simulink model "schema_simple"  (Simulink 7.0)
settings: Solver=ode5  SolverMode=SingleTasking  StartTime=0.0  StopTime=Inf  FixedStep=1e-3  MaxStep=0.001  RelTol=1e-3  AbsTol=1e-5
PreLoadFcn:
  | Ts=1e-3;
  | zdroj = 1;
  | man_w = 0.5
PostLoadFcn:
  | if ~exist('dsparch4','file') errordlg('Signal Processing Blockset is required to run this demo.', 'Signal Processing Blockset required'); end
undefined symbols (not defined in the file): Humusoft, MF624
libraries: rtwinlib x2
settings Model: Creator=Sehnal  SimulationMode=external  CovMetricSettings=d  ExtModeTrigDuration=50000  ExtModeTrigLevel=0.500000  ExtModeAutoUpdateStatusClock=off
settings SolverCC: PositivePriorityOrder=on
settings DataIOCC: LimitDataPoints=off  MaxDataPoints=10000  SaveOutput=off  SignalLogging=off  SaveTime=off  SignalLoggingName=logsOut
settings OptimizationCC: BooleanDataType=off
settings DebuggingCC: SaveWithParameterizedLinksMsg=none  CheckExecutionContextPreStartOutputMsg=on  CheckExecutionContextRuntimeOutputMsg=on  SignalResolutionControl=TryResolveAllWithWarning  SolverPrmCheckMsg=none  MultiTaskDSMMsg=warning  MultiTaskCondExecSysMsg=none  StrictBusMsg=None
settings HardwareCC: TargetEndianess=LittleEndian  TargetHWDeviceType=MATLAB Host  ProdEqTarget=off
settings ModelReferenceCC: UpdateModelReferenceTargets=IfOutOfDate  ModelReferenceNumInstancesAllowed=Zero
settings RTWCC: SystemTargetFile=rtwin.tlc  TemplateMakefile=rtwin.tmf  RetainRTWFile=on  ProcessScript=rtwin_make_rtw_hook  IncludeERTFirstTime=on
settings RTWinTargetCC: TargetFcnLib=ansi_tfl_tmw.mat  GenFloatMathFcnCalls=ANSI_C  ModelReferenceCompliant=off  CompOptLevelCompliant=off  PortableWordSizes=off  CCOptimize=on

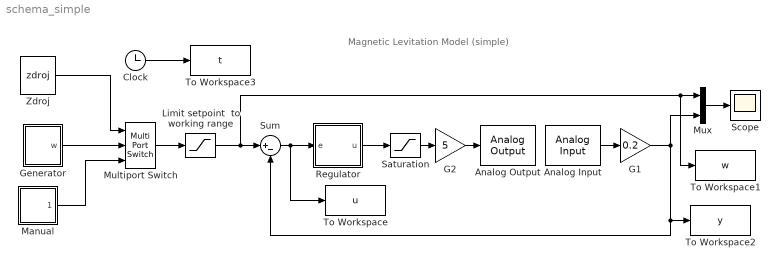
== system schema_simple ==
  note: Magnetic Levitation Model
      | (simple)
  Analog Input : rtwinlib/Analog Input  SampleTime=1e-3  DrvName=Humusoft/MF624  DrvAddress=4294967295  DrvOptions=0  Channels=1  RangeMode=1  VoltRange=1  DataType=1
      settings: AttributesFormatString=Humusoft\nMF624 [auto]
  Analog Output : rtwinlib/Analog Output  SampleTime=1e-3  DrvName=Humusoft/MF624  DrvAddress=4294967295  DrvOptions=0  Channels=1  RangeMode=1  VoltRange=1  InitialValue=0  FinalValue=0
      settings: AttributesFormatString=Humusoft\nMF624 [auto]
  Clock : Clock
      settings: Decimation=10
  G1 : Gain  Gain=0.2  ParameterDataType=sfix(16)  ParameterScaling=2^0  OutDataType=sfix(16)  OutScaling=2^0  SaturateOnIntegerOverflow=on
  G2 : Gain  Gain=5  ParameterDataType=sfix(16)  ParameterScaling=2^0  OutDataType=sfix(16)  OutScaling=2^0  SaturateOnIntegerOverflow=on
  Generator : Subsystem
  "Limit setpoint  to working range  " : Saturate  UpperLimit=0.8  LowerLimit=0  ZeroCross=off
  Manual : Subsystem
  Multiport Switch : MultiPortSwitch  Inputs=2
  Mux : Mux  Inputs=2
  Regulator : Subsystem
  Saturation : Saturate  UpperLimit=1  LowerLimit=0  ZeroCross=off
  Scope : Scope
      settings: TimeRange=5  YMin=-0.05  YMax=0.95  SaveName=last  DataFormat=Array  MaxDataPoints=1  SampleInput=on  SampleTime=0.02
  Sum : Sum  Inputs=|+-  OutDataType=sfix(16)  OutScaling=2^0  SaturateOnIntegerOverflow=on  InputSameDT=on
  To Workspace : ToWorkspace  VariableName=u  SampleTime=-1  SaveFormat=Array
  To Workspace1 : ToWorkspace  VariableName=w  SampleTime=-1  SaveFormat=Array
  To Workspace2 : ToWorkspace  VariableName=y  SampleTime=-1  SaveFormat=Array
  To Workspace3 : ToWorkspace  VariableName=t  SampleTime=-1  SaveFormat=Array
  Zdroj : Constant  Value=zdroj  OutDataType=sfix(16)  OutScaling=2^0
  wires:
  Sum/1 -> Regulator/1(e), To Workspace/1
  Analog Input/1 -> G1/1
  Saturation/1 -> G2/1
  G1/1 -> Mux/2, Sum/2, To Workspace2/1
  Zdroj/1 -> Multiport Switch/1
  Regulator/1(u) -> Saturation/1
  Generator/1(w) -> Multiport Switch/2
  Manual/1(man_w) -> Multiport Switch/3
  Multiport Switch/1 -> "Limit setpoint  to working range  "/1
  Mux/1 -> Scope/1
  G2/1 -> Analog Output/1
  "Limit setpoint  to working range  "/1 -> Sum/1, Mux/1, To Workspace1/1
  Clock/1 -> To Workspace3/1

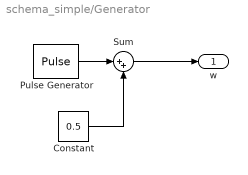
== system schema_simple/Generator ==
  Constant : Constant  Value=0.5  OutDataType=sfix(16)  OutScaling=2^0
  Pulse Generator : DiscretePulseGenerator  PulseType=Time based  Amplitude=0  Period=5  PulseWidth=50
  Sum : Sum  Inputs=|++  OutDataType=sfix(16)  OutScaling=2^0
  w : Outport  OutDataType=sfix(16)  OutScaling=2^0
  wires:
  Pulse Generator/1 -> Sum/1
  Constant/1 -> Sum/2
  Sum/1 -> w/1

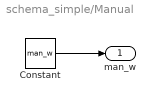
== system schema_simple/Manual ==
  Constant : Constant  Value=man_w  OutDataType=sfix(16)  OutScaling=2^0
  man_w : Outport  OutDataType=sfix(16)  OutScaling=2^0
  wires:
  Constant/1 -> man_w/1

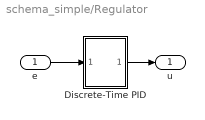
== system schema_simple/Regulator ==
  e : Inport  OutDataType=sfix(16)  OutScaling=2^0
  Discrete-Time PID : Subsystem  mask(PID){Kp=3, Ki=0.7, Kd=0.03, Ts=Ts}
      mask prompts: Ts "Sample time:"
      mask help: Discrete-time PID controller with limited integrator
      mask Display: disp('PID');
  u : Outport  OutDataType=sfix(16)  OutScaling=2^0
  wires:
  Discrete-Time PID/1(out_1) -> u/1
  e/1 -> Discrete-Time PID/1(in_1)

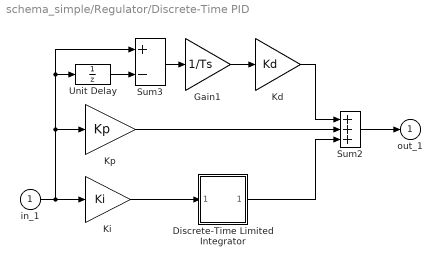
== system schema_simple/Regulator/Discrete-Time PID ==
  in_1 : Inport  OutDataType=sfix(16)  OutScaling=2^0
  Discrete-Time Limited Integrator : Subsystem  mask(Discrete-Time Limited Integrator.){@1=0, @2=2, @3=0, @4=Ts}
      mask prompts: @1 "Lower bound:"; @2 "Upper bound:"; @3 "Initial condition:"; @4 "Sampling Time:"
      mask help: Discrete-Time Limited Integrator.
      mask init:
      | lower_limit=@1;upper_limit=@2;X0=@3;Ts=@4;
      mask Help: Discrete-Time Limited Integrator. Unmask to see details.
      mask Display: plot(-1,-0.2,3.5,1.2,[0,1,2,2.9],[0,0,1,1],[0,1],[0.5,0.5], [.5,.5], [.8,.6], [.05,.35,.05,.35],[.4,.4,.2,.2], [.45,.65],[.3,.3], [.9,.9],[.2,.4]);
  Gain1 : Gain  Gain=1/Ts  ParameterDataType=sfix(16)  ParameterScaling=2^0  OutDataType=sfix(16)  OutScaling=2^0  SaturateOnIntegerOverflow=on
  Kd : Gain  Gain=Kd  ParameterDataType=sfix(16)  ParameterScaling=2^0  OutDataType=sfix(16)  OutScaling=2^0  SaturateOnIntegerOverflow=on
  Ki : Gain  Gain=Ki  ParameterDataType=sfix(16)  ParameterScaling=2^0  OutDataType=sfix(16)  OutScaling=2^0  SaturateOnIntegerOverflow=on
  Kp : Gain  Gain=Kp  ParameterDataType=sfix(16)  ParameterScaling=2^0  OutDataType=sfix(16)  OutScaling=2^0  SaturateOnIntegerOverflow=on
  Sum2 : Sum  Inputs=+++  OutDataType=sfix(16)  OutScaling=2^0  SaturateOnIntegerOverflow=on  InputSameDT=on
  Sum3 : Sum  Inputs=+-  OutDataType=sfix(16)  OutScaling=2^0  SaturateOnIntegerOverflow=on  InputSameDT=on
  Unit Delay : UnitDelay  SampleTime=Ts
  out_1 : Outport  OutDataType=sfix(16)  OutScaling=2^0  InitialOutput=0
  wires:
  Unit Delay/1 -> Sum3/2
  Kd/1 -> Sum2/1
  Kp/1 -> Sum2/2
  Sum2/1 -> out_1/1
  Sum3/1 -> Gain1/1
  Gain1/1 -> Kd/1
  in_1/1 -> Ki/1, Sum3/1, Unit Delay/1, Kp/1
  Ki/1 -> Discrete-Time Limited Integrator/1(in_1)
  Discrete-Time Limited Integrator/1(out_1) -> Sum2/3

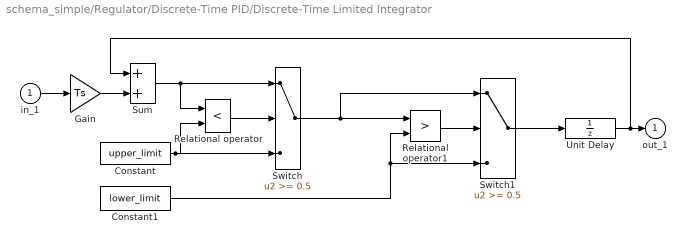
== system schema_simple/Regulator/Discrete-Time PID/Discrete-Time Limited Integrator ==
  in_1 : Inport  OutDataType=sfix(16)  OutScaling=2^0
  Constant : Constant  Value=upper_limit  OutDataType=sfix(16)  OutScaling=2^0
  Constant1 : Constant  Value=lower_limit  OutDataType=sfix(16)  OutScaling=2^0
  Gain : Gain  Gain=Ts  ParameterDataType=sfix(16)  ParameterScaling=2^0  OutDataType=sfix(16)  OutScaling=2^0  SaturateOnIntegerOverflow=on
  Relational operator : RelationalOperator  Operator=<  InputSameDT=on
  Relational operator1 : RelationalOperator  Operator=>  InputSameDT=on
  Sum : Sum  OutDataType=sfix(16)  OutScaling=2^0  SaturateOnIntegerOverflow=on  InputSameDT=on
  Switch : Switch  Threshold=0.5  InputSameDT=on
  Switch1 : Switch  Threshold=0.5  InputSameDT=on
  Unit Delay : UnitDelay  X0=X0  SampleTime=Ts
  out_1 : Outport  OutDataType=sfix(16)  OutScaling=2^0  InitialOutput=0
  wires:
  Unit Delay/1 -> out_1/1, Sum/1
  Switch1/1 -> Unit Delay/1
  Constant1/1 -> Relational operator1/2, Switch1/3
  Relational operator1/1 -> Switch1/2
  Switch/1 -> Relational operator1/1, Switch1/1
  Constant/1 -> Switch/3, Relational operator/2
  Gain/1 -> Sum/2
  Sum/1 -> Switch/1, Relational operator/1
  Relational operator/1 -> Switch/2
  in_1/1 -> Gain/1
